simulink model "P3Simulink"  (R2024a)
settings: Solver=VariableStepAuto  StartTime=0.0  StopTime=5  RelTol=1e-3
InitFcn:
  | m1=290;
  | b1=1000;
  | m2=59;
  | k1=16182;
  | f=0;
  | k2=19000;
settings Model: Creator=Becho  LastModifiedBy=Becho

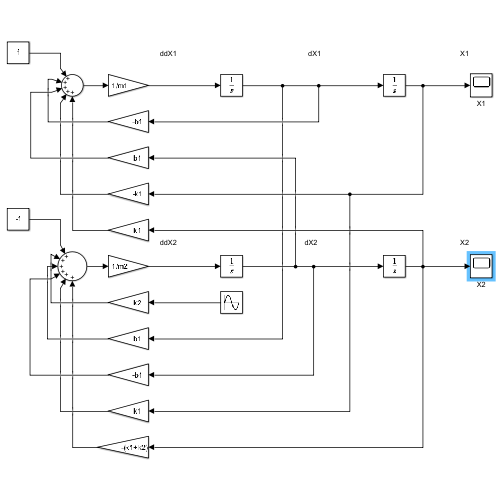
[thumbnail: Simulink's stored preview of the top-level diagram]
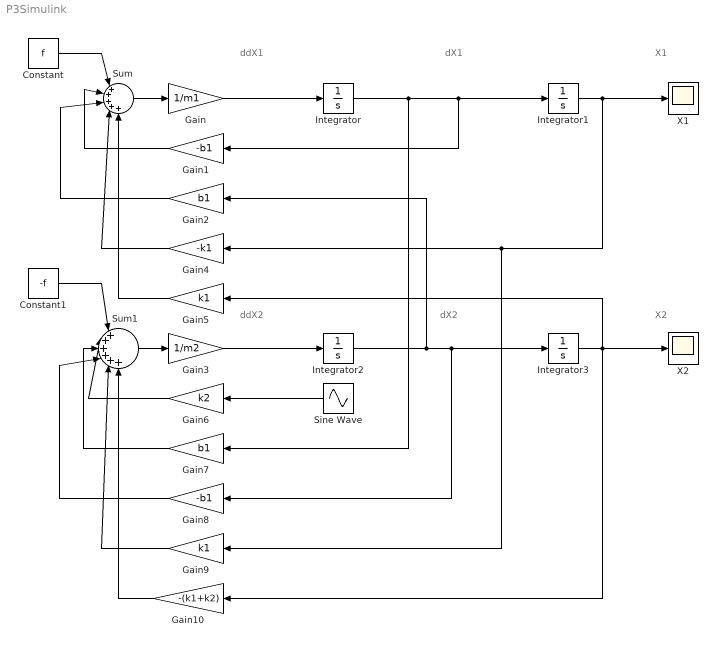
== system P3Simulink ==
  note: ddX1
  note: dX1
  note: X1
  note: ddX2
  note: dX2
  note: X2
  Constant : Constant  Value=f
  Constant1 : Constant  Value=-f
  Gain : Gain  Gain=1/m1
  Gain1 : Gain  Gain=-b1
  Gain10 : Gain  Gain=-(k1+k2)
  Gain2 : Gain  Gain=b1
  Gain3 : Gain  Gain=1/m2
  Gain4 : Gain  Gain=-k1
  Gain5 : Gain  Gain=k1
  Gain6 : Gain  Gain=k2
  Gain7 : Gain  Gain=b1
  Gain8 : Gain  Gain=-b1
  Gain9 : Gain  Gain=k1
  Integrator{,1..3} (4 alike) : Integrator
  Sine Wave : Sin  Amplitude=.05  Frequency=.5*pi  SampleTime=0
  Sum : Sum  Inputs=|+++++
  Sum1 : Sum  Inputs=|++++++
  X1 : Scope
  X2 : Scope
  wires:
  Integrator/1 -> Gain7/1, Gain1/1, Integrator1/1
  Gain/1 -> Integrator/1
  Sum/1 -> Gain/1
  Constant/1 -> Sum/1
  Gain1/1 -> Sum/2
  Sum1/1 -> Gain3/1
  Gain3/1 -> Integrator2/1
  Integrator2/1 -> Gain2/1, Gain8/1, Integrator3/1
  Gain2/1 -> Sum/3
  Integrator1/1 -> X1/1, Gain9/1, Gain4/1
  Gain4/1 -> Sum/4
  Integrator3/1 -> X2/1, Gain5/1, Gain10/1
  Gain5/1 -> Sum/5
  Constant1/1 -> Sum1/1
  Sine Wave/1 -> Gain6/1
  Gain6/1 -> Sum1/2
  Gain7/1 -> Sum1/3
  Gain8/1 -> Sum1/4
  Gain9/1 -> Sum1/5
  Gain10/1 -> Sum1/6
